simulink model "PendulumRobot"  (R2023b)
settings: Solver=FixedStepDiscrete  StartTime=0.0  StopTime=30  FixedStep=Ts  RelTol=1e-3  EnableMultiTasking=on
values from neighbouring files (symbols this model uses):
  A = [0 1 0 0; 0 a_11 a_13 0; 0 0 0 1; 0 a_41 a_43 0]    [initializeRobot.m]
  B = [0; b_1; 0; b_4]    [initializeRobot.m]
  C = [1 0 0 0; 0 1 0 0; 0 0 1 0; 0 0 0 1]    [initializeRobot.m]
  D = [0; 0; 0; 0]    [initializeRobot.m]
  K = place(A,B,e)    [initializeRobot.m]
  N = [0 0 0 0; 0 0 0 0; 0 0 0 0; 0 0 0 0]    [initializeRobot.m]
  R = [r1 0 0 0; 0 r2 0 0; 0 0 r3 0; 0 0 0 r4]    [initializeRobot.m]
  r = 0.034    [initializeRobot.m]
  ref = [0; 0; -(pi/180)*4; 0]    [initializeRobot.m]
  T_filt = 0.01    [initializeRobot.m]
  Ts = 0.01    [initializeRobot.m]
  x0 = [0; 0; (pi/180)*10; 0]    [initializeRobot.m]
undefined symbols (not defined in the file or in its folder): DiscIntNeverNeededParam, Discrete, Time
libraries: cstblocks x2, ctrlSharedLib x1, arduinosensorlib x1, SpeedEstimater x1, TB6612FNG x1
settings Model: ExtModeTrigDuration=2  Creator=user  LastModifiedBy=user
settings OptimizationCC: EnhancedBackFolding=on  PassReuseOutputArgsAs=Individual arguments  ZeroExternalMemoryAtStartup=off  ZeroInternalMemoryAtStartup=off  MaxStackSize=64  OptimizeBlockOrder=speed  DifferentSizesBufferReuse=on  OptimizationCustomize=off  EfficientTunableParamExpr=on
settings DebuggingCC: ParameterPrecisionLossMsg=none  ParameterTunabilityLossMsg=error
settings HardwareCC: ProdBitPerInt=16  ProdBitPerPointer=16  ProdBitPerSizeT=16  ProdBitPerPtrDiffT=16  ProdWordSize=8  ProdHWDeviceType=Atmel->AVR  UseEmbeddedCoderFeatures=off  UseSimulinkCoderFeatures=off
settings SFSimCC: MATLABDynamicMemAlloc=off
settings RTWCC: Description=Embedded Coder  SystemTargetFile=ert.tlc  HardwareBoard=Arduino Uno  TemplateMakefile=ert_default_tmf  Toolchain=Arduino AVR  BuildConfiguration=Faster Runs
settings CodeAppCC: ForceParamTrailComments=on  IgnoreCustomStorageClasses=off  OperatorAnnotations=on  SimulinkDataObjDesc=on  SFDataObjDesc=on  InsertBlockDesc=on
settings ERTTargetCC: SupportContinuousTime=on  SupportNonInlinedSFcns=on  SupportVariableSizeSignals=on  ExtModeTransport=3  ExtModeStaticAlloc=on  ExtModeAutomaticAllocSize=off  ExtModeStaticAllocSize=250  ExtModeMexFile=ext_xcp  ExtModeIntrfLevel=Level2 - Open

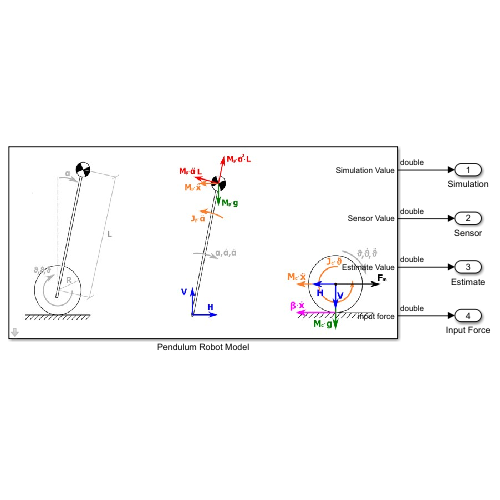
[thumbnail: Simulink's stored preview of the top-level diagram]
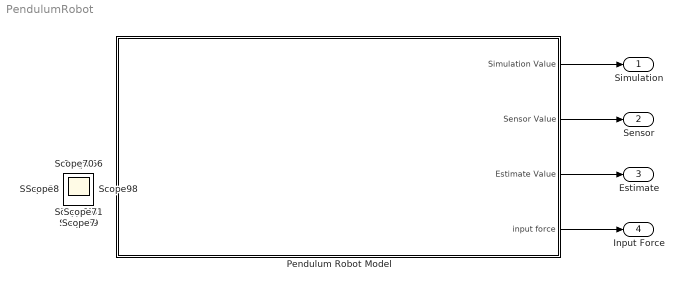
== system PendulumRobot ==
  Pendulum Robot Model : Subsystem  InitFcn=[Ts, T_filt, r, ref, x0, A, B, C, D, K, P0, Q, R, N] = initializeRobot()  mask{K=K, A=A, B=B, C=C, D=D}
      mask prompts: K "制御ゲイン K："; A "システム行列 A："; B "入力係数行列 B："; C "観測行列 C："; D "直達行列 D："
      mask DialogControl Container1 Prompt: 状態空間表現
      mask DialogControl Control1 Prompt: 各パラメータの詳細は初期化関数で定義
      mask DialogControl Container2 Prompt: 状態方程式：x_dot = Ax + Bu
      mask DialogControl Container3 Prompt: 出力方程式：x_dot = Cx + Du
      mask DialogControl Container4 Prompt: 制御パラメータ
      mask Display: image('PendulumRobotModel.jpg');
  Simulation : Outport
  Sensor : Outport  Port=2
  Estimate : Outport  Port=3
  Input Force : Outport  Port=4
  Scope{,1..71} (72 alike) : Scope
  wires:
  Pendulum Robot Model/1(Simulation Value) -> Simulation/1
  Pendulum Robot Model/2(Sensor Value) -> Sensor/1
  Pendulum Robot Model/3(Estimate Value) -> Estimate/1
  Pendulum Robot Model/4(input force) -> Input Force/1

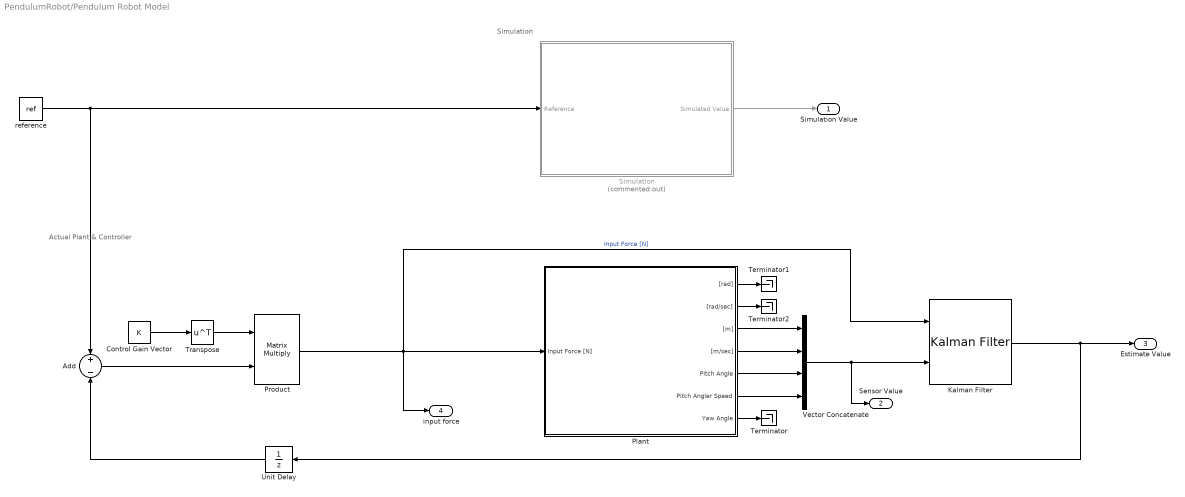
== system PendulumRobot/Pendulum Robot Model ==
  note: Actual Plant & Controller
  note: Simulation
  Add : Sum  Inputs=+-
  Control Gain Vector : Constant  Value=K
  Kalman Filter : ctrlSharedLib/Kalman Filter  TimeDomain=Discrete-Time  UseCurrentEstimator=on  ModelSource=Individual A, B, C, D matrices  ModelSourceVariable=ss(A,B,C,D)  A=A  B=B  C=C  D=D  NumberOfStates=1  NumberOfInputs=1  NumberOfOutputs=1  InitialEstimateSource=Dialog  X0=x0  P0=10  UseK=off  UseGH=off  NumberOfProcessNoiseInputs=1  G=1  TimeInvariantG=on  H=0  TimeInvariantH=on  Q=Q  TimeInvariantQ=on  R=R  TimeInvariantR=on  N=N  TimeInvariantN=on  AddInputPort=on  AddEnablePort=off  OutputEstimatedY=off  OutputP=off  Ts=-1
  Plant : Subsystem  mask{T_filt=T_filt, Kt=0.011, Vec=5, Res=6.28, r=r, pulse=1560}
      mask prompts: T_filt "ローパスフィルタのカットオフ周波数 T_filt [sec]："; Kt "トルク定数 Kt [N·m/A]："; Vec "回路の供給電圧 Vec [V]："; Res "モータの抵抗 Res [Ω]："; r "タイヤ半径[m]："; pulse "モータが1回転するときのパルス数："
      mask TypeOptions pulse: Speed Estimate/pulse
      mask DialogControl Container1 Prompt: 実機パラメータ
      mask Display: image('Elegoo_Tumbller.jpeg');
  Product : Product  Multiplication=Matrix(*)
  Simulation : Subsystem  Commented=on
  Terminator : Terminator
  Terminator1 : Terminator
  Terminator2 : Terminator
  Transpose : Math  Operator=transpose
  Unit Delay : UnitDelay  SampleTime=-1  HasFrameUpgradeWarning=on
  Vector Concatenate : Concatenate  NumInputs=4
  reference : Constant  Value=ref  SampleTime=Ts
  Simulation Value : Outport
  Sensor Value : Outport  Port=2
  Estimate Value : Outport  Port=3
  input force : Outport  Port=4
  wires:
  Plant/6(Pitch Angler Speed) -> Vector Concatenate/4
  Product/1 -> Plant/1(Input Force [N]), Kalman Filter/1, input force/1  "Input Force [N]"
  Plant/7(Yaw Angle) -> Terminator/1
  Plant/5(Pitch Angle) -> Vector Concatenate/3
  Kalman Filter/1 -> Unit Delay/1, Estimate Value/1
  Control Gain Vector/1 -> Transpose/1
  reference/1 -> Add/1, Simulation/1(Reference)
  Simulation/1(Simulated Value) -> Simulation Value/1
  Transpose/1 -> Product/1
  Vector Concatenate/1 -> Kalman Filter/2, Sensor Value/1
  Add/1 -> Product/2
  Plant/1("[rad]") -> Terminator1/1
  Plant/2("[rad/sec]") -> Terminator2/1
  Plant/4("[m/sec]") -> Vector Concatenate/2
  Plant/3("[m]") -> Vector Concatenate/1
  Unit Delay/1 -> Add/2

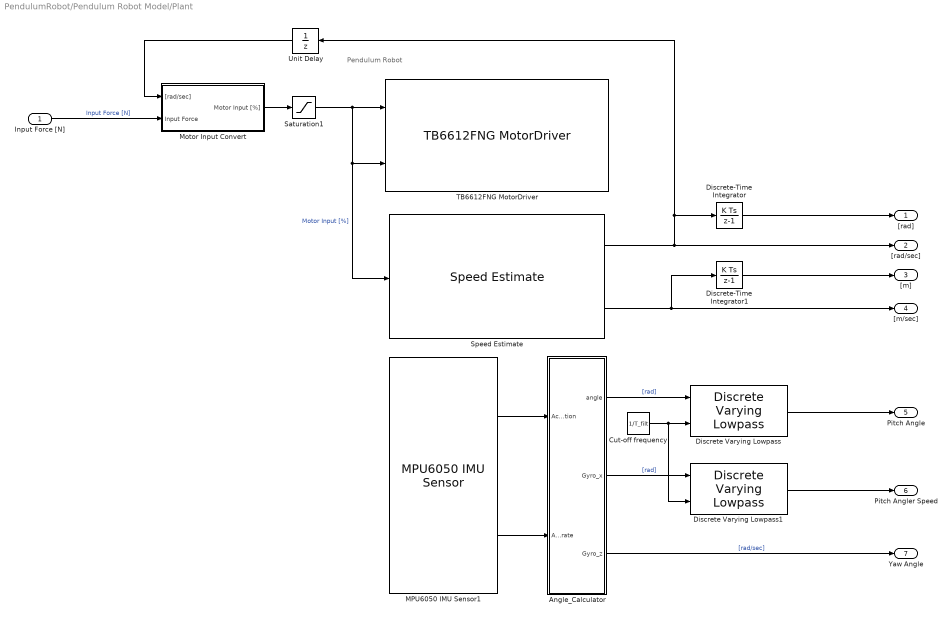
== system PendulumRobot/Pendulum Robot Model/Plant ==
  note: Pendulum Robot
  Input Force [N] : Inport
  Angle_Calculator : Subsystem
  Cut-off frequency : Constant  Value=1/T_filt
  Discrete Varying Lowpass : cstblocks/Linear Parameter Varying/Discrete Varying Lowpass  N=1  w0=0  Ts=Ts
  Discrete Varying Lowpass1 : cstblocks/Linear Parameter Varying/Discrete Varying Lowpass  N=1  w0=0  Ts=Ts
  Discrete-Time Integrator : DiscreteIntegrator  SampleTime=-1  ICPrevOutput=DiscIntNeverNeededParam  ICPrevScaledInput=DiscIntNeverNeededParam
  Discrete-Time Integrator1 : DiscreteIntegrator  SampleTime=-1  ICPrevOutput=DiscIntNeverNeededParam  ICPrevScaledInput=DiscIntNeverNeededParam
  MPU6050 IMU Sensor1 : arduinosensorlib/MPU6050 IMU Sensor  SlaveAddress=0x68  Accel=on  AngularRate=on  Temperature=off  Status=off  Timestamp=off  EulerAngles=off  Quat=off  AccelRange=2G  GyroRange=250 dps  DmpOdr=200 Hz  Dlpf=Accelerometer: 184Hz, Gyroscope: 188Hz  spf=1  SampleTime=-1  QueueSizeFactor=1
  Motor Input Convert : Subsystem  mask{Kt=Kt, Vec=Vec, Res=Res, r=r}
      mask prompts: Kt "トルク定数 Kt [N·m/A]："; Vec "回路の供給電圧 Vmax [V]："; Res "モータの抵抗 Res [Ω]："; r "タイヤ半径 r [m]："
      mask DialogControl ParameterGroupVar Prompt: Parameter
  Saturation1 : Saturate  UpperLimit=100  LowerLimit=-100
  Speed Estimate : SpeedEstimater/Speed Estimate  pinExt=2  pinA=4  r=r  Ts=Ts  pulse=pulse
  TB6612FNG MotorDriver : TB6612FNG/TB6612FNG MotorDriver  SetBYPin=8  InputAPin=7  EnablePin1=5  InputBPin=12  EnablePin2=6
  Unit Delay : UnitDelay  SampleTime=-1  HasFrameUpgradeWarning=on
  "[rad]" : Outport
  "[rad/sec]" : Outport  Port=2
  "[m]" : Outport  Port=3
  "[m/sec]" : Outport  Port=4
  Pitch Angle : Outport  Port=5
  Pitch Angler Speed : Outport  Port=6
  Yaw Angle : Outport  Port=7
  wires:
  MPU6050 IMU Sensor1/2 -> Angle_Calculator/2(Anglar rate)
  Angle_Calculator/3(Gyro_z) -> Yaw Angle/1  "[rad/sec]"
  Motor Input Convert/1(Motor Input [%]) -> Saturation1/1
  Input Force [N]/1 -> Motor Input Convert/2(Input Force)  "Input Force [N]"
  Saturation1/1 -> Speed Estimate/1, TB6612FNG MotorDriver/2, TB6612FNG MotorDriver/1  "Motor Input [%]"
  Angle_Calculator/1(angle) -> Discrete Varying Lowpass/1  "[rad]"
  Discrete Varying Lowpass/1 -> Pitch Angle/1
  Angle_Calculator/2(Gyro_x) -> Discrete Varying Lowpass1/1  "[rad]"
  Cut-off frequency/1 -> Discrete Varying Lowpass1/2, Discrete Varying Lowpass/2
  Discrete Varying Lowpass1/1 -> Pitch Angler Speed/1
  MPU6050 IMU Sensor1/1 -> Angle_Calculator/1(Acceleration)
  Speed Estimate/2 -> Discrete-Time Integrator1/1, "[m/sec]"/1
  Speed Estimate/1 -> Unit Delay/1, Discrete-Time Integrator/1, "[rad/sec]"/1
  Discrete-Time Integrator/1 -> "[rad]"/1
  Discrete-Time Integrator1/1 -> "[m]"/1
  Unit Delay/1 -> Motor Input Convert/1("[rad/sec]")

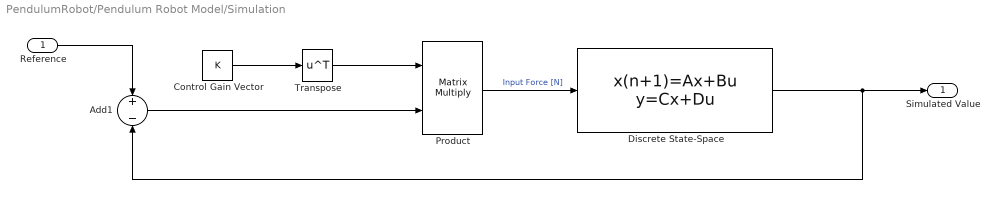
== system PendulumRobot/Pendulum Robot Model/Simulation ==
  Reference : Inport
  Add1 : Sum  Inputs=+-
  Control Gain Vector : Constant  Value=K
  Discrete State-Space : DiscreteStateSpace  A=A  B=B  C=C  D=D  InitialCondition=x0  SampleTime=-1
  Product : Product  Multiplication=Matrix(*)
  Transpose : Math  Operator=transpose
  Simulated Value : Outport
  wires:
  Reference/1 -> Add1/1
  Discrete State-Space/1 -> Simulated Value/1, Add1/2
  Add1/1 -> Product/2
  Transpose/1 -> Product/1
  Control Gain Vector/1 -> Transpose/1
  Product/1 -> Discrete State-Space/1  "Input Force [N]"

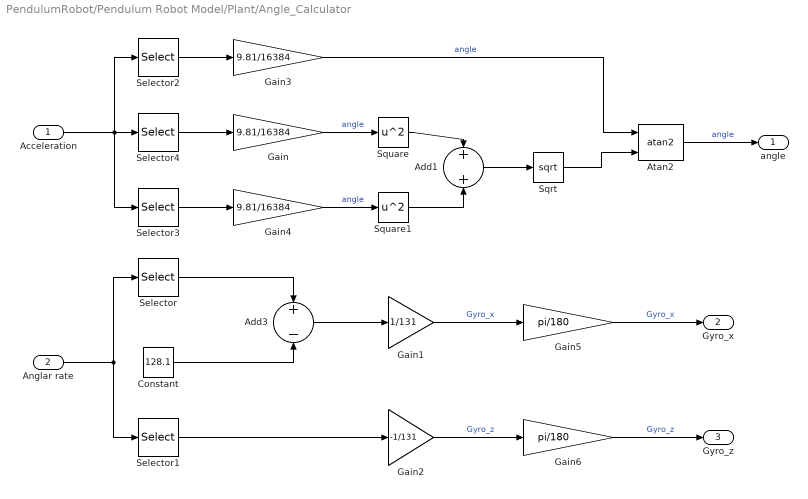
== system PendulumRobot/Pendulum Robot Model/Plant/Angle_Calculator ==
  Acceleration : Inport
  Anglar rate : Inport  Port=2
  Add1 : Sum
  Add3 : Sum  Inputs=+-
  Atan2 : Trigonometry  Operator=atan2
  Constant : Constant  Value=128.1
  Gain : Gain  Gain=9.81/16384
  Gain1 : Gain  Gain=1/131
  Gain2 : Gain  Gain=-1/131
  Gain3 : Gain  Gain=9.81/16384
  Gain4 : Gain  Gain=9.81/16384
  Gain5 : Gain  Gain=pi/180
  Gain6 : Gain  Gain=pi/180
  Selector : Selector  InputPortWidth=3  IndexOptions=Index vector (dialog)  Indices=[1]  OutputSizes=1
  Selector1 : Selector  InputPortWidth=3  IndexOptions=Index vector (dialog)  Indices=[3]  OutputSizes=1
  Selector2 : Selector  InputPortWidth=3  IndexOptions=Index vector (dialog)  Indices=[2]  OutputSizes=1
  Selector3 : Selector  InputPortWidth=3  IndexOptions=Index vector (dialog)  Indices=[3]  OutputSizes=1
  Selector4 : Selector  InputPortWidth=3  IndexOptions=Index vector (dialog)  Indices=[1]  OutputSizes=1
  Sqrt : Sqrt
  Square : Math  Operator=square
  Square1 : Math  Operator=square
  angle : Outport
  Gyro_x : Outport  Port=2
  Gyro_z : Outport  Port=3
  wires:
  Acceleration/1 -> Selector4/1, Selector2/1, Selector3/1
  Anglar rate/1 -> Selector1/1, Selector/1
  Selector/1 -> Add3/1
  Selector2/1 -> Gain3/1
  Constant/1 -> Add3/2
  Add3/1 -> Gain1/1
  Gain1/1 -> Gain5/1  "Gyro_x"
  Selector1/1 -> Gain2/1
  Gain2/1 -> Gain6/1  "Gyro_z"
  Selector4/1 -> Gain/1
  Gain3/1 -> Atan2/1  "angle"
  Selector3/1 -> Gain4/1
  Gain/1 -> Square/1  "angle"
  Gain4/1 -> Square1/1  "angle"
  Square1/1 -> Add1/2
  Square/1 -> Add1/1
  Add1/1 -> Sqrt/1
  Sqrt/1 -> Atan2/2
  Atan2/1 -> angle/1  "angle"
  Gain5/1 -> Gyro_x/1  "Gyro_x"
  Gain6/1 -> Gyro_z/1  "Gyro_z"

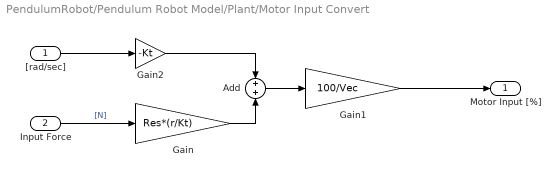
== system PendulumRobot/Pendulum Robot Model/Plant/Motor Input Convert ==
  "[rad/sec]" : Inport
  Input Force : Inport  Port=2
  Add : Sum
  Gain : Gain  Gain=Res*(r/Kt)
  Gain1 : Gain  Gain=100/Vec
  Gain2 : Gain  Gain=-Kt
  Motor Input [%] : Outport
  wires:
  Input Force/1 -> Gain/1  "[N]"
  Gain1/1 -> Motor Input [%]/1
  Gain/1 -> Add/2
  Add/1 -> Gain1/1
  "[rad/sec]"/1 -> Gain2/1
  Gain2/1 -> Add/1
